simulink model "pitchShift"  (R2022a)
settings: Solver=VariableStepAuto  StartTime=0.0  StopTime=3  RelTol=1e-3
PostLoadFcn:
  | postLoadCallback
InitFcn:
  | initCallback
StopFcn:
  | stopCallback
undefined symbols (not defined in the file): modelParams
libraries: hdlsllib x6, dspsrcs4 x2
CloseFcn:
  | closeCallback
settings Model: Creator=Ronnel  LastModifiedBy=Ronnel
settings DataIOCC: ReturnWorkspaceOutputs=off
settings OptimizationCC: BlockReduction=off  ConditionallyExecuteInputs=off  DefaultParameterBehavior=Inlined
settings DebuggingCC: AlgebraicLoopMsg=error
settings HardwareCC: ProdBitPerPointer=32  ProdBitPerSizeT=32  ProdBitPerPtrDiffT=32  ProdLargestAtomicFloat=None  ProdIntDivRoundTo=Undefined  ProdEndianess=Unspecified  ProdWordSize=32  ProdHWDeviceType=ASIC/FPGA->ASIC/FPGA  TargetBitPerPointer=64  TargetBitPerSizeT=64  TargetBitPerPtrDiffT=64  TargetLongLongMode=on  TargetIntDivRoundTo=Zero  TargetEndianess=LittleEndian  TargetWordSize=64  TargetHWDeviceType=Custom Processor->MATLAB Host Computer  ProdEqTarget=off

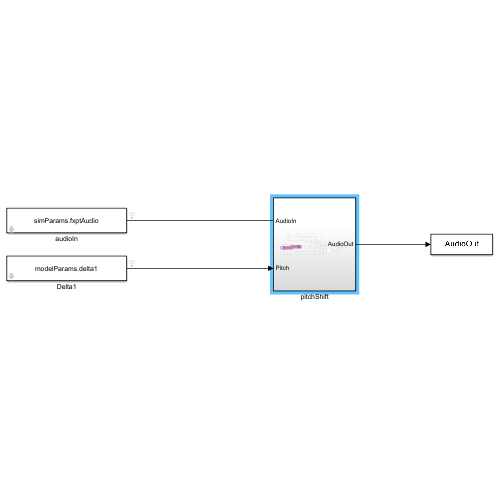
[thumbnail: Simulink's stored preview of the top-level diagram]
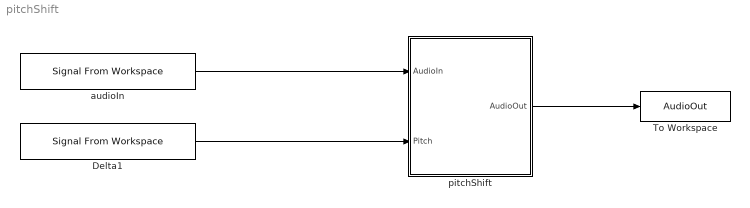
== system pitchShift ==
  Delta1 : dspsrcs4/Signal From Workspace  X=modelParams.delta1  Ts=modelParams.audio.samplePeriod  nsamps=1  OutputAfterFinalValue=Setting to zero  ignoreOrWarnInputAndFrameLengths=off  OutputFrames=off
  To Workspace : ToWorkspace  VariableName=AudioOut  SampleTime=-1
  audioIn : dspsrcs4/Signal From Workspace  X=simParams.fxptAudio  Ts=modelParams.audio.samplePeriod  nsamps=1  OutputAfterFinalValue=Setting to zero  ignoreOrWarnInputAndFrameLengths=off  OutputFrames=off
  pitchShift : Subsystem
  wires:
  audioIn/1 -> pitchShift/1(AudioIn)
  pitchShift/1(AudioOut) -> To Workspace/1
  Delta1/1 -> pitchShift/2(Pitch)

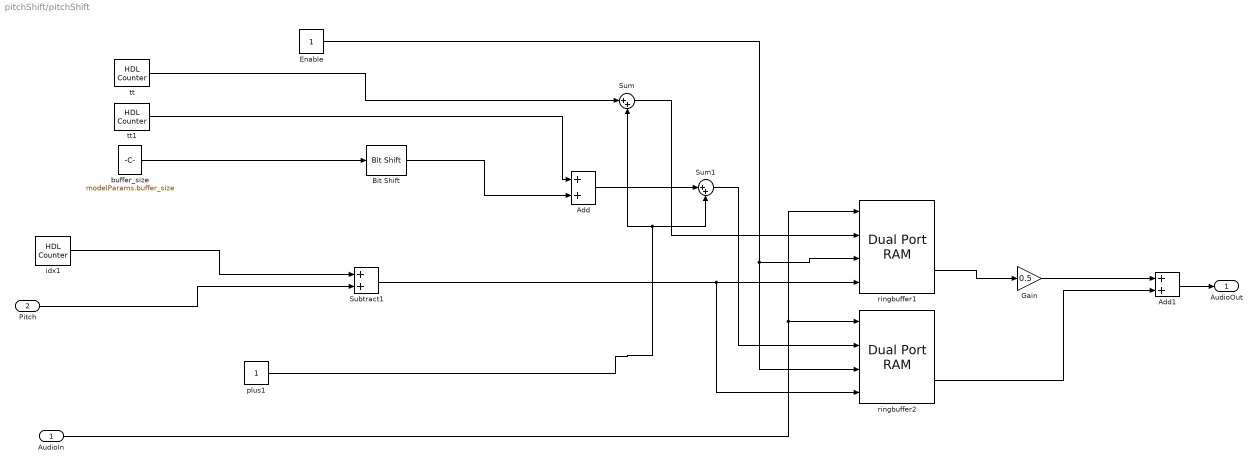
== system pitchShift/pitchShift ==
  AudioIn : Inport  SampleTime=modelParams.audio.samplePeriod
  Pitch : Inport  Port=2  SampleTime=modelParams.audio.samplePeriod
  Add : Sum  SampleTime=modelParams.audio.samplePeriod
  Add1 : Sum  OutDataTypeStr=fixdt(1,24,16)  SampleTime=modelParams.audio.samplePeriod
  Bit Shift : hdlsllib/Logic and Bit Operations/Bit Shift  mode=Shift Right Logical  N=1
  Enable : Constant  OutDataTypeStr=boolean  SampleTime=modelParams.audio.samplePeriod
  Gain : Gain  Gain=0.5  SampleTime=modelParams.audio.samplePeriod
  Subtract1 : Sum  OutDataTypeStr=Inherit: Inherit via back propagation  RndMeth=Round  SampleTime=modelParams.audio.samplePeriod
  Sum : Sum  Inputs=|++  OutDataTypeStr=uint16  SampleTime=modelParams.audio.samplePeriod
  Sum1 : Sum  Inputs=|++  OutDataTypeStr=uint16  SampleTime=modelParams.audio.samplePeriod
  buffer_size : Constant  Value=modelParams.buffer_size  SampleTime=modelParams.audio.samplePeriod
  idx1 : hdlsllib/Sources/HDL Counter  CountType=Free running  CountInit=0  CountStep=1  CountMax=25  CountFromType=Initial value  CountFrom=0  CountResetPort=off  CountLoadPort=off  CountEnbPort=off  CountDirPort=off  CountHitOutputPort=off  CountDataType=Unsigned  CountWordLen=modelParams.dpramAddressSize + modelParams.audio.fractionLength  CountFracLen=modelParams.audio.fractionLength  CountSampTime=modelParams.audio.samplePeriod
  plus1 : Constant  OutDataTypeStr=Inherit: Inherit via back propagation  SampleTime=modelParams.audio.samplePeriod
  ringbuffer1 : hdlsllib/HDL RAMs/Dual Port RAM  ram_size=16
      settings: SourceProductBaseCode=SL
  ringbuffer2 : hdlsllib/HDL RAMs/Dual Port RAM  ram_size=16
      settings: SourceProductBaseCode=SL
  tt : hdlsllib/Sources/HDL Counter  CountType=Free running  CountInit=1  CountStep=1  CountMax=25  CountFromType=Initial value  CountFrom=1  CountResetPort=off  CountLoadPort=off  CountEnbPort=off  CountDirPort=off  CountHitOutputPort=off  CountDataType=Unsigned  CountWordLen=modelParams.dpramAddressSize  CountFracLen=0  CountSampTime=modelParams.audio.samplePeriod
  tt1 : hdlsllib/Sources/HDL Counter  CountType=Free running  CountInit=1  CountStep=1  CountMax=25  CountFromType=Initial value  CountFrom=1  CountResetPort=off  CountLoadPort=off  CountEnbPort=off  CountDirPort=off  CountHitOutputPort=off  CountDataType=Unsigned  CountWordLen=modelParams.dpramAddressSize-1  CountFracLen=0  CountSampTime=modelParams.audio.samplePeriod
  AudioOut : Outport
  wires:
  Bit Shift/1 -> Add/2
  ringbuffer2/2 -> Add1/2
  Enable/1 -> ringbuffer2/3, ringbuffer1/3
  Add/1 -> Sum1/1
  AudioIn/1 -> ringbuffer2/1, ringbuffer1/1
  buffer_size/1 -> Bit Shift/1
  ringbuffer1/2 -> Gain/1
  tt/1 -> Sum/1
  Gain/1 -> Add1/1
  plus1/1 -> Sum/2, Sum1/2
  Sum/1 -> ringbuffer1/2
  Sum1/1 -> ringbuffer2/2
  Subtract1/1 -> ringbuffer1/4, ringbuffer2/4
  Add1/1 -> AudioOut/1
  tt1/1 -> Add/1
  Pitch/1 -> Subtract1/2
  idx1/1 -> Subtract1/1
